simulink model "navigator"  (R2021a)
settings: Solver=FixedStepAuto  StartTime=0.0  StopTime=10.0  FixedStep=0.05  RelTol=1e-3
undefined symbols (not defined in the file): CONSTANTS_RADIUS_OF_EARTH, GF_ACTION, GF_MAX_HOR_DIST, GF_MAX_VER_DIST
(part 1 of 3)
settings Model: DataDictionary=px4_dict.sldd  Creator=DELL  LastModifiedBy=DELL

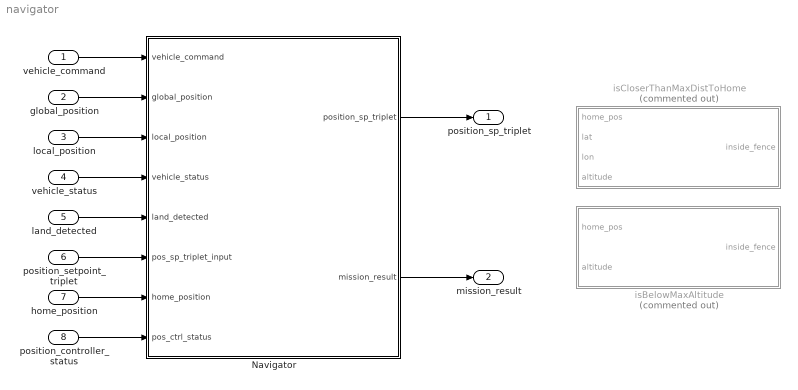
== system navigator ==
  vehicle_command : Inport  OutDataTypeStr=Bus: px4_vehicle_command
  global_position : Inport  Port=2  OutDataTypeStr=Bus: px4_vehicle_global_position
  local_position : Inport  Port=3  OutDataTypeStr=Bus: px4_vehicle_local_position
  vehicle_status : Inport  Port=4  OutDataTypeStr=Bus: px4_vehicle_status
  land_detected : Inport  Port=5  OutDataTypeStr=Bus: px4_vehicle_land_detected
  position_setpoint_triplet : Inport  Port=6  OutDataTypeStr=Bus: px4_position_setpoint_triplet
  home_position : Inport  Port=7  OutDataTypeStr=Bus: px4_home_position
  position_controller_status : Inport  Port=8  OutDataTypeStr=Bus: px4_position_controller_status
  Navigator : Stateflow chart  TreatAsAtomicUnit=on
  isBelowMaxAltitude : MATLAB Function  Commented=on  TreatAsAtomicUnit=on
  isCloserThanMaxDistToHome : MATLAB Function  Commented=on  TreatAsAtomicUnit=on
  position_sp_triplet : Outport
  mission_result : Outport  Port=2
  wires:
  vehicle_command/1 -> Navigator/1(vehicle_command)
  global_position/1 -> Navigator/2(global_position)
  local_position/1 -> Navigator/3(local_position)
  vehicle_status/1 -> Navigator/4(vehicle_status)
  land_detected/1 -> Navigator/5(land_detected)
  position_setpoint_triplet/1 -> Navigator/6(pos_sp_triplet_input)
  home_position/1 -> Navigator/7(home_position)
  position_controller_status/1 -> Navigator/8(pos_ctrl_status)
  Navigator/1(position_sp_triplet) -> position_sp_triplet/1
  Navigator/2(mission_result) -> mission_result/1
